simulink model "hand"  (R2024b)
settings: Solver=FixedStepAuto  StartTime=0.0  StopTime=inf  FixedStep=0.001  RelTol=1e-3
undefined symbols (not defined in the file or in its folder): X, Y, Z
libraries: sm_lib x122, nesl_utility x36, simulink x1
(part 2 of 2)

== matlab function hand/Forward Kinematics ==
  data: thumb_o output; index_o output; middle_o output; ring_o output; pinky_o output; x input
function [thumb_o,index_o,middle_o,ring_o,pinky_o] = fingerKinematicsAll(x)
    % MATLAB Function to compute the forward kinematics of all fingers
    % Output:
    % T_all - A struct containing 4x4 transformation matrices for each finger

    % Define Transformation Functions
    function T = transX(d)
        T = [1 0 0 d; 0 1 0 0; 0 0 1 0; 0 0 0 1];
    end

    function T = transY(d)
        T = [1 0 0 0; 0 1 0 d; 0 0 1 0; 0 0 0 1];
    end

    function T = transZ(d)
        T = [1 0 0 0; 0 1 0 0; 0 0 1 d; 0 0 0 1];
    end

    function T = rotX(theta)
        T = [1 0 0 0; 0 cosd(theta) -sind(theta) 0; 0 sind(theta) cosd(theta) 0; 0 0 0 1];
    end

    function T = rotY(theta)
        T = [cosd(theta) 0 sind(theta) 0; 0 1 0 0; -sind(theta) 0 cosd(theta) 0; 0 0 0 1];
    end

    function T = rotZ(theta)
        T = [cosd(theta) -sind(theta) 0 0; sind(theta) cosd(theta) 0 0; 0 0 1 0; 0 0 0 1];
    end

    % Predefined Joint Angles for Each Finger (Assumed)
    angles.thumb  = [x(1,1), x(2,1), x(3,1)];  % Thumb joint angles
    angles.index  = [x(1,2), x(2,2), x(3,2)];  % Index Finger joint angles
    angles.middle = [x(1,3), x(2,3), x(3,3)];  % Middle Finger joint angles
    angles.ring  = [x(1,4), x(2,4), x(3,4)];  % Pinky Finger joint angles
    angles.pinky   = [x(1,5), x(2,5), x(3,5)];  % Ring Finger joint angles

    % Define Finger-Specific Transformations
    % middle = rotY(90) * transY(1.1) * rotZ(90) * rotZ(angles.middle(1)) * transX(1) * rotZ(angles.middle(2)) * transX(1) * rotZ(angles.middle(3)) * transX(1);
    % 
    % index = transX(-0.6) * rotY(90) * transY(1) * rotZ(90) * rotZ(angles.index(1)) * transX(1) * rotZ(angles.index(2)) * transX(1) * rotZ(angles.index(3)) * transX(1);
    % 
    % ring = transX(0.6) * rotY(90) * transY(1) * rotZ(90) * rotZ(angles.ring(1)) * transX(1) * rotZ(angles.ring(2)) * transX(1) * rotZ(angles.ring(3)) * transX(1);
    % 
    % pinky = transX(1.2) * rotY(90) * transY(0.4) * rotZ(90) * rotZ(angles.pinky(1)) * transX(1) * rotZ(angles.pinky(2)) * transX(1) * rotZ(angles.pinky(3))  * transX(1);
    % 
    % thumb = transX(-0.6) * rotZ(60) * rotY(90)  * transY(0.8) * rotZ(90) * rotZ(angles.thumb(1)) * transX(0.6) * rotZ(angles.thumb(2)) * transX(0.6) * rotZ(angles.thumb(3))  * transX(0.6);

    middle = rotZ(angles.middle(1)) * transX(1) * rotZ(angles.middle(2)) * transX(1) * rotZ(angles.middle(3)) * transX(1);
               
    index = rotZ(angles.index(1)) * transX(1) * rotZ(angles.index(2)) * transX(1) * rotZ(angles.index(3)) * transX(1);

    ring = rotZ(angles.ring(1)) * transX(1) * rotZ(angles.ring(2)) * transX(1) * rotZ(angles.ring(3)) * transX(1);

    pinky = rotZ(angles.pinky(1)) * transX(1) * rotZ(angles.pinky(2)) * transX(1) * rotZ(angles.pinky(3))  * transX(1);

    thumb = rotZ(angles.thumb(1)) * transX(0.6) * rotZ(angles.thumb(2)) * transX(0.6) * rotZ(angles.thumb(3))  * transX(0.6);

    middle_o = middle(1:3,4);
    index_o  = index(1:3,4);
    ring_o   = ring(1:3,4);
    pinky_o  = pinky(1:3,4);
    thumb_o  = thumb(1:3,4);
end

== matlab function hand/MATLAB Function1 ==
  data: end_effector input; q output
function q = fcn(end_effector)
    % ข้อมูลความยาวของลิงก์ (5 หุ่นยนต์)
    L = [0.6, 0.6, 0.6; 
         1, 1, 1; 
         1, 1, 1; 
         1, 1, 1; 
         1, 1, 1];

    % ตรวจสอบว่าข้อมูลอินพุตมีขนาด 4x5 หรือไม่
    if size(end_effector, 1) ~= 4 || size(end_effector, 2) ~= 5
        error('Input must be a 4x5 array (x, y, z, theta for 5 robots)');
    end

    % เตรียมพื้นที่สำหรับผลลัพธ์ (q1, q2, q3 สำหรับหุ่นยนต์ 5 ตัว)
    q = zeros(3, 5);

    % วนลูปคำนวณ Inverse Kinematics สำหรับหุ่นยนต์แต่ละตัว
    for i = 1:size(end_effector, 2)
        % ดึงข้อมูล x, y, z, theta จาก end_effector
        x = end_effector(1, i);
        y = end_effector(2, i);
        z = end_effector(3, i);
        theta = end_effector(4, i);

        % คำนวณตำแหน่งข้อมือ (wrist center) ในระนาบเฉียง
        x_wrist = x - L(i,3) * sin(theta);
        y_wrist = y - L(i,3) * cos(theta);

        % คำนวณระยะ r จากฐานถึงข้อมือ
        r = sqrt(x_wrist^2 + y_wrist^2);

        % ตรวจสอบ workspace
        min_reach = abs(L(i,1) - L(i,2)); % ระยะขั้นต่ำที่แขนสามารถเอื้อมถึง
        max_reach = L(i,1) + L(i,2);      % ระยะสูงสุดที่แขนสามารถเอื้อมถึง

        if r - min_reach < 0.001 || max_reach - r > 0.001
            warning('Target position is out of reach for robot %d. Skipping this calculation.', i);
            q(:, i) = NaN; % กำหนดค่า NaN สำหรับหุ่นยนต์ที่ไม่สามารถคำนวณได้
            continue;
        end

        % คำนวณ cos(q2)
        cos_q2 = (r^2 - L(i,1)^2 - L(i,2)^2) / (2 * L(i,1) * L(i,2));

        % ตรวจสอบว่าค่า cos(q2) อยู่ในช่วงที่ยอมรับได้
        if cos_q2 < -1 || cos_q2 > 1
            warning('Cosine value out of range for robot %d. Skipping this calculation.', i);
            q(:, i) = NaN; % กำหนดค่า NaN สำหรับหุ่นยนต์ที่ไม่สามารถคำนวณได้
            continue;
        end

        % คำนวณ q2
        q2 = acos(cos_q2);

        % คำนวณ q1
        beta = atan2(L(i,2) * sin(q2), L(i,1) + L(i,2) * cos(q2));
        alpha = atan2(y_wrist, x_wrist); % มุมจากฐานถึงตำแหน่งข้อมือ
        q1 = alpha - beta;

        % คำนวณ q3
        q3 = theta - q1 - q2;

        % จัดเก็บผลลัพธ์ใน q
        q(:, i) = [q1; q2; q3];

    end
end

== matlab function hand/Plant/MATLAB Function ==
  data: u input; o1 output; o2 output; o3 output; o4 output; o5 output; o6 output; o7 output; o8 output; o9 output; o10 output; o11 output; o12 output; o13 output; o14 output; o15 output
function [o1, o2, o3,o4, o5, o6, o7, o8, o9, o10, o11, o12, o13, o14, o15] = fcn(u)
    o1 = u(1, 1);
    o2 = u(2, 1);
    o3 = u(3, 1);
    o4 = u(1, 2);
    o5 = u(2, 2);
    o6 = u(3, 2);
    o7 = u(1, 3);
    o8 = u(2, 3);
    o9 = u(3, 3);
    o10 = u(1, 4);
    o11 = u(2, 4);
    o12 = u(3, 4);
    o13 = u(1, 5);
    o14 = u(2, 5);
    o15 = u(3, 5);

== matlab function hand/Quintic Trajectory ==
  data: target_q1 input; q output; button_state input; t input
function q = fcn(target_q1, button_state, t)
    % กำหนดตัวแปร persistent
    persistent curr_q t_start run_started a0 a1 a2 a3 a4 a5
    
    [rows, cols] = size(target_q1); % ตรวจสอบขนาดของ input
    if isempty(curr_q)
        % กำหนดค่าเริ่มต้นให้กับ curr_q เป็น array ขนาด [3xN]
        curr_q = zeros(rows, cols);
        t_start = 0;
        run_started = 0;
        
        % กำหนดค่าเริ่มต้นให้กับ coefficients
        a0 = zeros(rows, cols);
        a1 = zeros(rows, cols);
        a2 = zeros(rows, cols);
        a3 = zeros(rows, cols);
        a4 = zeros(rows, cols);
        a5 = zeros(rows, cols);
    end

    % ตรวจสอบให้แน่ใจว่า target_q1 มีขนาด [3xN]
    if size(target_q1, 1) ~= 3
        disp(size(target_q1))
        % error('target_q1 ต้องเป็น array ขนาด [3xN]');
    end

    tf = 5; % กำหนดเวลาสิ้นสุดของ trajectory

    % เริ่มต้นการทำงานเมื่อ button_state เป็น 1
    if button_state == 1 && run_started == 0
        run_started = 1;
        t_start = t;
        
        % คำนวณ delta_q สำหรับแต่ละ element
        delta_q = target_q1 - curr_q;
        
        % คำนวณ coefficients สำหรับ quintic polynomial trajectory
        a0 = curr_q;
        a1 = zeros(rows, cols);
        a2 = zeros(rows, cols);
        a3 = 10 * delta_q / (tf^3);
        a4 = -15 * delta_q / (tf^4);
        a5 = 6 * delta_q / (tf^5);
    end

    % คำนวณ trajectory
    q = curr_q; % ค่าเริ่มต้นของ q
    if run_started == 1
        elapsed_time = t - t_start;
        if elapsed_time <= tf
            % คำนวณ q ตาม quintic trajectory
            q = a0 + a1 * elapsed_time + a2 * (elapsed_time^2) + ...
                a3 * (elapsed_time^3) + a4 * (elapsed_time^4) + a5 * (elapsed_time^5);
        else
            % เมื่อถึงเวลาสิ้นสุด ให้ q เท่ากับ target
            q = target_q1;
            run_started = 0;
        end
        % อัพเดตค่า current q
        curr_q = q;
    end
end

== matlab function hand/Input/MATLAB Function ==
  data: i input; o1 output; o2 output; o3 output; o4 output; o5 output; o6 output; o7 output; o8 output; o9 output; o10 output; o11 output; o12 output; o13 output; o14 output; o15 output
function [o1, o2, o3,o4, o5, o6, o7, o8, o9, o10, o11, o12, o13, o14, o15] = fcn(i)
    if i(1) == 1
        o1 = 90;
        o2 = 90;
        o3 = 90;
    else
        o1 = 0;
        o2 = 0;
        o3 = 0; 
    end

    if i(2) == 1
        o4 = 90;
        o5 = 90;
        o6 = 90;
    else
        o4 = 0;
        o5 = 0;
        o6 = 0; 
    end

    if i(3) == 1
        o7 = 90;
        o8 = 90;
        o9 = 90;
    else
        o7 = 0;
        o8 = 0;
        o9 = 0; 
    end

    if i(4) == 1
        o10 = 90;
        o11 = 90;
        o12 = 90;
    else
        o10 = 0;
        o11 = 0;
        o12 = 0; 
    end

    if i(5) == 1
        o13 = 90;
        o14 = 90;
        o15 = 90;
    else
        o13 = 0;
        o14 = 0;
        o15 = 0; 
    end

== matlab function hand/Plant/MATLAB Function1 ==
  data: x output; transSig input; y output; z output
function [x, y, z] = getPosition(transSig)
x = transSig(1);
y = transSig(2);
z = transSig(3);
end

== matlab function hand/MATLAB Function ==
  data: chk_collision input; q output; button_state input; flag output
function [q, flag]= fcn(chk_collision, button_state)
    % กำหนดตัวแปร persistent
    persistent curr_q run_started stop_columns

    [rows, cols] = size(chk_collision); % ตรวจสอบขนาดของ input
    if isempty(curr_q)
        % กำหนดค่าเริ่มต้นให้กับ curr_q เป็น array ขนาด [rows x cols]
        curr_q = zeros(rows, cols);
        run_started = 0;
        stop_columns = false(rows, cols); % ติดตามสถานะการชนแต่ละแถว-คอลัมน์
        
    end

    flag = 0;

    % เริ่มต้นการทำงานเมื่อ button_state เป็น 1
    if button_state == 1 && run_started == 0
        run_started = 1;
    end

    % คำนวณ trajectory
    q = curr_q; % ค่าเริ่มต้นของ q
    if run_started == 1
        for i = 1:rows
            for j = 1:cols
                if stop_columns(i, j)
                    % หากหยุดการเพิ่มค่าของคอลัมน์ j ในแถว i
                    q(i, j) = curr_q(i, j);
                elseif i == 1 && chk_collision(i, j) == 0
                    % แถวแรก เพิ่มค่าเสมอ
                    q(i, j) = curr_q(i, j) + 0.02;
                elseif chk_collision(i, j) == 1
                    % เมื่อชนในแถว i คอลัมน์ j
                    % 1. หยุดเพิ่มในแถวก่อนหน้า (1 ถึง i)
                    stop_columns(1:i, j) = true;
                elseif stop_columns(i-1, j)
                    q(i, j) = curr_q(i, j) + 0.02;
                else
                    % ไม่ชนและไม่ถูกหยุดเพิ่ม
                    q(i, j) = curr_q(i, j);
                end
            end
        end
        curr_q = q; % อัปเดตตำแหน่งปัจจุบัน
    end

    if all(stop_columns == 1)
        flag = 1;
    end
end

== matlab function hand/Plant/MATLAB Function2 ==
  data: x output; transSig input; y output; z output
function [x, y, z] = getPosition(transSig)
x = transSig(1);
y = transSig(2);
z = transSig(3);
end

== matlab function hand/Plant/MATLAB Function3 ==
  data: x output; transSig input; y output; z output
function [x, y, z] = getPosition(transSig)
x = transSig(1);
y = transSig(2);
z = transSig(3);
end
